simulink model "voltage_to_kelvin"  (R2020b)
settings: Solver=ode45  StartTime=0.0  StopTime=10.0  RelTol=1e-3  EnableMultiTasking=on
settings Model: Creator=USER  LastModifiedBy=USER
settings DataIOCC: LimitDataPoints=on  SaveFormat=Array  ReturnWorkspaceOutputs=off
settings OptimizationCC: LifeSpan=inf
settings DebuggingCC: SFUnexpectedBacktrackingDiag=warning  SFNoUnconditionalDefaultTransitionDiag=warning  SFExecutionAtInitializationDiag=none  ArithmeticOperatorsInVariantConditions=warning
settings HardwareCC: ProdBitPerPointer=32  ProdBitPerSizeT=32  ProdBitPerPtrDiffT=32  ProdLargestAtomicFloat=None  ProdIntDivRoundTo=Undefined  ProdEndianess=Unspecified  ProdWordSize=32  ProdHWDeviceType=32-bit Generic
settings ModelReferenceCC: PropagateSignalLabelsOutOfModel=off
settings SFSimCC: SimUseLocalCustomCode=off  CustomCodeUndefinedFunction=UseInterfaceOnly
settings RTWCC: RTWUseLocalCustomCode=off
settings CodeAppCC: StateflowObjectComments=on
settings GRTTargetCC: TargetLangStandard=C89/C90 (ANSI)
settings ConfigComp: CovMetricSettings=dw  CovSaveCumulativeToWorkspaceVar=on  CovSaveSingleToWorkspaceVar=on  CovExternalEMLEnable=off

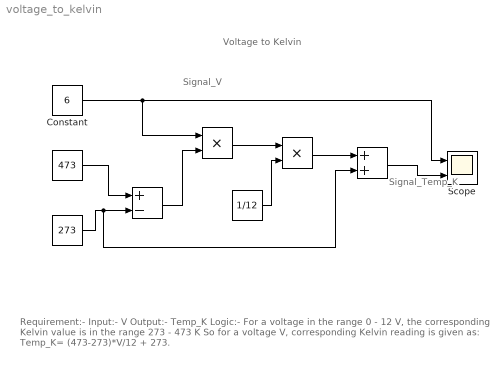
== system voltage_to_kelvin ==
  note: Signal_V
  note: Signal_Temp_K
  note: Requirement:-
      |
      | Input:- V
      | Output:- Temp_K
      | Logic:- For a voltage in the range 0 - 12 V, the corresponding Kelvin value is in the range 273 - 473 K
      | 	     So for a voltage V, corresponding Kelvin reading is given as:
      | 	     Temp_K= (473-273)*V/12 + 273.
  note: Voltage to Kelvin
  " " : Constant  Value=473
  "  " : Constant  Value=273
  "   " : Constant  Value=1/12
  "    " : Product
  "     " : Sum  Inputs=+-
  "      " : Sum
  "       " : Product
  Constant : Constant  Value=6
  Scope : Scope  NumInputPorts=2
  wires:
  " "/1 -> "     "/1
  "  "/1 -> "      "/2, "     "/2
  Constant/1 -> Scope/1, "    "/1
  "     "/1 -> "    "/2
  "    "/1 -> "       "/1
  "   "/1 -> "       "/2
  "       "/1 -> "      "/1
  "      "/1 -> Scope/2
